simulink model "control_layer_ZMP_COM"  (Simulink 7.9)
settings: Solver=ode45  StartTime=0.0  StopTime=10.0  RelTol=1e-3
values from neighbouring files (symbols this model uses):
  k1 = -q(1)*q(2)-1    [WPG_results.m]    (also in WPG_results_10.m; WPG_results_2.m; WPG_results_3.m; WPG_results_4.m)
  k2 = (q(1)+q(2))/-q(3)    [WPG_results.m]    (also in WPG_results_10.m; WPG_results_2.m; WPG_results_3.m; WPG_results_4.m)
  k3 = w    [WPG_results.m]    (also in WPG_results_10.m; WPG_results_2.m; WPG_results_3.m; WPG_results_4.m)
settings Model: Creator=pajon  LastModifiedBy=pajon

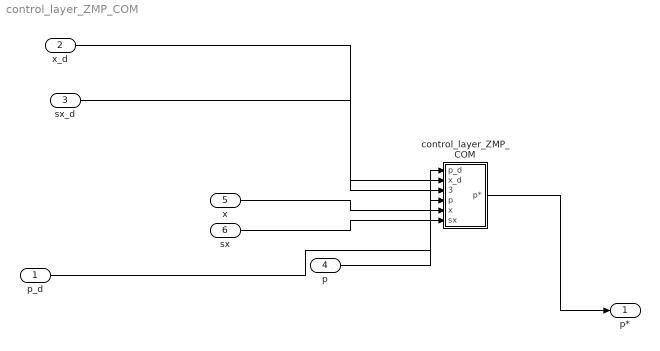
== system control_layer_ZMP_COM ==
  p_d : Inport
  x_d : Inport  Port=2
  sx_d : Inport  Port=3
  p : Inport  Port=4
  x : Inport  Port=5
  sx : Inport  Port=6
  control_layer_ZMP_COM : Subsystem
  p* : Outport
  wires:
  p_d/1 -> control_layer_ZMP_COM/1(p_d)
  x_d/1 -> control_layer_ZMP_COM/2(x_d)
  sx_d/1 -> control_layer_ZMP_COM/3(sx_d)
  p/1 -> control_layer_ZMP_COM/4(p)
  x/1 -> control_layer_ZMP_COM/5(x)
  sx/1 -> control_layer_ZMP_COM/6(sx)
  control_layer_ZMP_COM/1(p*) -> p*/1

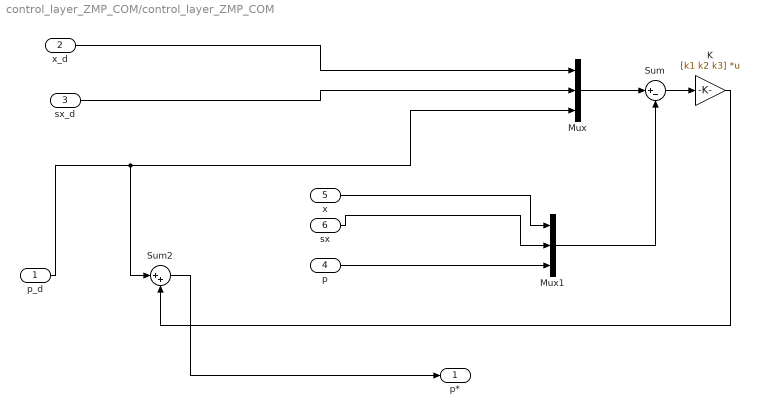
== system control_layer_ZMP_COM/control_layer_ZMP_COM ==
  p_d : Inport
  x_d : Inport  Port=2
  sx_d : Inport  Port=3
  p : Inport  Port=4
  x : Inport  Port=5
  sx : Inport  Port=6
  K : Gain  Gain=[k1 k2 k3]  Multiplication=Matrix(K*u)
  Mux : Mux  Inputs=3
  Mux1 : Mux  Inputs=3
  Sum : Sum  Inputs=|+-
  Sum2 : Sum  Inputs=|++
  p* : Outport
  wires:
  Mux/1 -> Sum/1
  Mux1/1 -> Sum/2
  Sum/1 -> K/1
  K/1 -> Sum2/2
  Sum2/1 -> p*/1
  x/1 -> Mux1/1
  sx/1 -> Mux1/2
  p_d/1 -> Mux/3, Sum2/1
  x_d/1 -> Mux/1
  sx_d/1 -> Mux/2
  p/1 -> Mux1/3
